simulink model "Quadcopter_CTC_Quaternion_Control"  (R2025a)
settings: Solver=FixedStepAuto  StartTime=0  StopTime=30  FixedStep=step_size  RelTol=1e-5
values from neighbouring files (symbols this model uses):
  g = 9.81    [Parameters.m]
  mQ = 1.5    [Parameters.m]
libraries: aerolibutil x1, sharedutil x1, slpidlib x1
settings Model: Creator=Mohamed Eid  LastModifiedBy=HP
settings DataIOCC: SaveFormat=StructureWithTime
settings OptimizationCC: BlockReduction=off  BufferReuse=off
settings DebuggingCC: SignalInfNanChecking=error  AlgebraicLoopMsg=none
settings ModelReferenceCC: EnableRefExpFcnMdlSchedulingChecks=on
settings RTWCC: GPUComputeCapability=3.5  DLArmComputeVersion=19.05

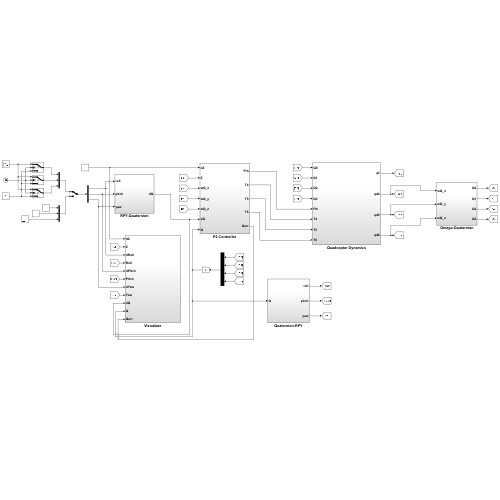
[thumbnail: Simulink's stored preview of the top-level diagram]
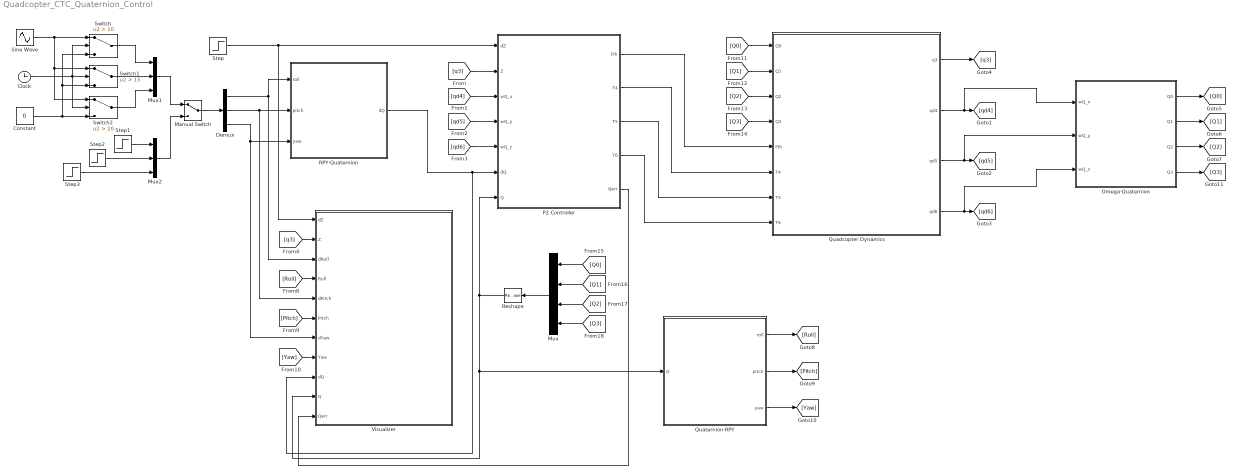
== system Quadcopter_CTC_Quaternion_Control ==
  Clock : Clock
  Constant : Constant  Value=0
  Demux : Demux  Outputs=3
  Manual Switch : ManualSwitch
  Mux : Mux
  Mux1 : Mux  Inputs=3
  Mux2 : Mux  Inputs=3
  Omega-Quaternion : Subsystem
  P2 Controller : Subsystem
  Quadcopter Dynamics : Subsystem
  Quaternion-RPY : Subsystem
  RPY-Quaternion : Subsystem
  Reshape : Reshape  OutputDimensionality=Customize  OutputDimensions=[4,1]
  Sine Wave : Sin  Amplitude=0.5  Frequency=2*pi/5  SampleTime=0
  Step : Step  After=10  SampleTime=0
  Step1 : Step  Time=10  After=30*pi/180  SampleTime=0
  Step2 : Step  Time=15  After=30*pi/180  SampleTime=0
  Step3 : Step  Time=20  After=30*pi/180  SampleTime=0
  Switch : Switch  Criteria=u2 > Threshold  Threshold=10  SaturateOnIntegerOverflow=off  InputSameDT=off
  Switch1 : Switch  Criteria=u2 > Threshold  Threshold=15  SaturateOnIntegerOverflow=off  InputSameDT=off
  Switch2 : Switch  Criteria=u2 > Threshold  Threshold=20  SaturateOnIntegerOverflow=off  InputSameDT=off
  Visualizer : Subsystem
  wires:
  Demux/2 -> Visualizer/5(dPitch), RPY-Quaternion/2(pitch)
  Quadcopter Dynamics/4(qd6) -> Omega-Quaternion/3(wQ_z), [qd6]
  Demux/1 -> RPY-Quaternion/1(roll), Visualizer/3(dRoll)
  Quadcopter Dynamics/2(qd4) -> Omega-Quaternion/1(wQ_x), [qd4]
  Quadcopter Dynamics/3(qd5) -> Omega-Quaternion/2(wQ_y), [qd5]
  Demux/3 -> Visualizer/7(dYaw), RPY-Quaternion/3(yaw)
  Quadcopter Dynamics/1(q3) -> [q3]
  [q3] -> P2 Controller/2(Z)
  [qd6] -> P2 Controller/5(wQ_z)
  [qd5] -> P2 Controller/4(wQ_y)
  [qd4] -> P2 Controller/3(wQ_x)
  Step/1 -> Visualizer/1(dZ), P2 Controller/1(dZ)
  RPY-Quaternion/1(dQ) -> Visualizer/9(dQ), P2 Controller/6(dQ)
  [q3] -> Visualizer/2(Z)
  Mux/1 -> Reshape/1
  Quaternion-RPY/2(pitch) -> [Pitch]
  Quaternion-RPY/1(roll) -> [Roll]
  Quaternion-RPY/3(yaw) -> [Yaw]
  [Roll] -> Visualizer/4(Roll)
  [Pitch] -> Visualizer/6(Pitch)
  [Yaw] -> Visualizer/8(Yaw)
  Reshape/1 -> P2 Controller/7(Q), Visualizer/10(Q), Quaternion-RPY/1(Q)
  P2 Controller/4(T6) -> Quadcopter Dynamics/8(T6)
  P2 Controller/3(T5) -> Quadcopter Dynamics/7(T5)
  P2 Controller/2(T4) -> Quadcopter Dynamics/6(T4)
  P2 Controller/1(Fth) -> Quadcopter Dynamics/5(Fth)
  P2 Controller/5(Qerr) -> Visualizer/11(Qerr)
  Omega-Quaternion/1(Q0) -> [Q0]
  Omega-Quaternion/2(Q1) -> [Q1]
  Omega-Quaternion/3(Q2) -> [Q2]
  Omega-Quaternion/4(Q3) -> [Q3]
  [Q0] -> Quadcopter Dynamics/1(Q0)
  [Q1] -> Quadcopter Dynamics/2(Q1)
  [Q2] -> Quadcopter Dynamics/3(Q2)
  [Q3] -> Quadcopter Dynamics/4(Q3)
  [Q0] -> Mux/1
  [Q1] -> Mux/2
  [Q2] -> Mux/3
  [Q3] -> Mux/4
  Constant/1 -> Switch/3, Switch1/3, Switch2/3
  Sine Wave/1 -> Switch2/1, Switch1/1, Switch/1
  Clock/1 -> Switch2/2, Switch/2, Switch1/2
  Step1/1 -> Mux2/1
  Step2/1 -> Mux2/2
  Step3/1 -> Mux2/3
  Switch1/1 -> Mux1/2
  Switch/1 -> Mux1/1
  Switch2/1 -> Mux1/3
  Manual Switch/1 -> Demux/1
  Mux1/1 -> Manual Switch/1
  Mux2/1 -> Manual Switch/2

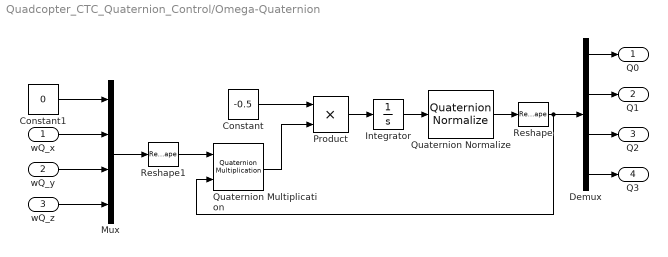
== system Quadcopter_CTC_Quaternion_Control/Omega-Quaternion ==
  wQ_x : Inport
  wQ_y : Inport  Port=2
  wQ_z : Inport  Port=3
  Constant : Constant  Value=-0.5
  Constant1 : Constant  Value=0
  Demux : Demux
  Integrator : Integrator  InitialCondition=[1;0;0;0]
  Mux : Mux
  Product : Product
  Quaternion Multiplication : aerolibutil/Quaternion Multiplication
  Quaternion Normalize : sharedutil/Quaternion Normalize  aMode=aMode
  Reshape : Reshape  OutputDimensionality=Customize  OutputDimensions=[4,1]
  Reshape1 : Reshape  OutputDimensionality=Customize  OutputDimensions=[4,1]
  Q0 : Outport
  Q1 : Outport  Port=2
  Q2 : Outport  Port=3
  Q3 : Outport  Port=4
  wires:
  Integrator/1 -> Quaternion Normalize/1
  Quaternion Normalize/1 -> Reshape/1
  Reshape/1 -> Quaternion Multiplication/2, Demux/1
  Demux/4 -> Q3/1
  Demux/3 -> Q2/1
  Demux/2 -> Q1/1
  Demux/1 -> Q0/1
  Constant/1 -> Product/1
  Quaternion Multiplication/1 -> Product/2
  Product/1 -> Integrator/1
  wQ_z/1 -> Mux/4
  wQ_y/1 -> Mux/3
  wQ_x/1 -> Mux/2
  Constant1/1 -> Mux/1
  Mux/1 -> Reshape1/1
  Reshape1/1 -> Quaternion Multiplication/1

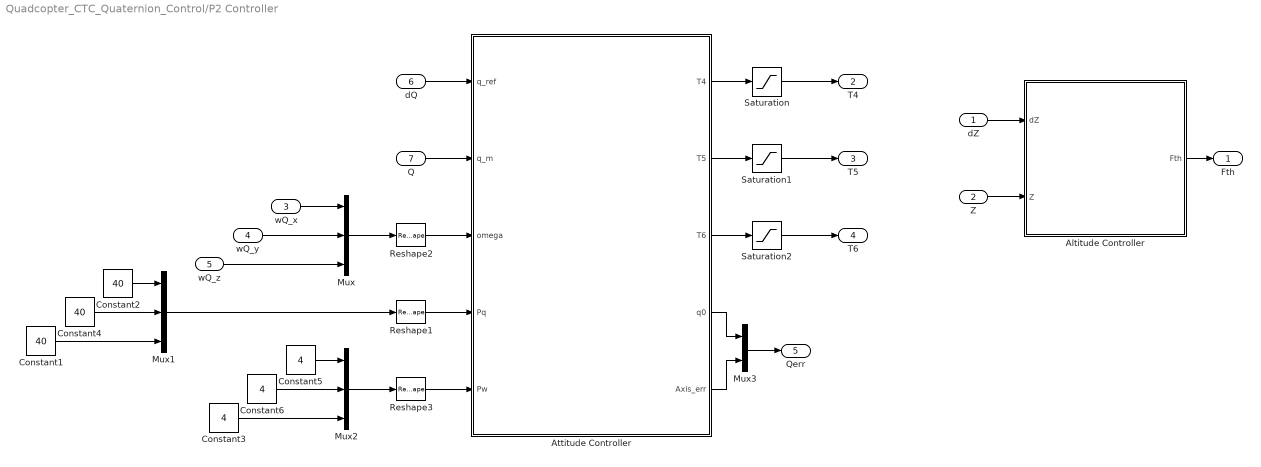
== system Quadcopter_CTC_Quaternion_Control/P2 Controller ==
  dZ : Inport
  Z : Inport  Port=2
  wQ_x : Inport  Port=3
  wQ_y : Inport  Port=4
  wQ_z : Inport  Port=5
  dQ : Inport  Port=6
  Q : Inport  Port=7
  Altitude Controller : Subsystem
  Attitude Controller : MATLAB Function  TreatAsAtomicUnit=on
  Constant1 : Constant  Value=40
  Constant2 : Constant  Value=40
  Constant3 : Constant  Value=4
  Constant4 : Constant  Value=40
  Constant5 : Constant  Value=4
  Constant6 : Constant  Value=4
  Mux : Mux  Inputs=3
  Mux1 : Mux  Inputs=3
  Mux2 : Mux  Inputs=3
  Mux3 : Mux  Inputs=2
  Reshape1 : Reshape  OutputDimensionality=Customize  OutputDimensions=[1,3]
  Reshape2 : Reshape  OutputDimensionality=Customize  OutputDimensions=[3,1]
  Reshape3 : Reshape  OutputDimensionality=Customize  OutputDimensions=[1,3]
  Saturation : Saturate  UpperLimit=1.842326154870013  LowerLimit=-1.842326154870013
  Saturation1 : Saturate  UpperLimit=1.842326154870013  LowerLimit=-1.842326154870013
  Saturation2 : Saturate  UpperLimit=0.104069495295931  LowerLimit=-0.104069495295931
  Fth : Outport
  T4 : Outport  Port=2
  T5 : Outport  Port=3
  T6 : Outport  Port=4
  Qerr : Outport  Port=5
  wires:
  Mux/1 -> Reshape2/1
  wQ_x/1 -> Mux/1
  wQ_y/1 -> Mux/2
  wQ_z/1 -> Mux/3
  Attitude Controller/1(T4) -> Saturation/1
  dZ/1 -> Altitude Controller/1(dZ)
  Z/1 -> Altitude Controller/2(Z)
  Altitude Controller/1(Fth) -> Fth/1
  dQ/1 -> Attitude Controller/1(q_ref)
  Q/1 -> Attitude Controller/2(q_m)
  Reshape2/1 -> Attitude Controller/3(omega)
  Mux3/1 -> Qerr/1
  Attitude Controller/2(T5) -> Saturation1/1
  Attitude Controller/3(T6) -> Saturation2/1
  Attitude Controller/4(q0) -> Mux3/1
  Attitude Controller/5(Axis_err) -> Mux3/2
  Saturation/1 -> T4/1
  Saturation1/1 -> T5/1
  Saturation2/1 -> T6/1
  Constant4/1 -> Mux1/2
  Mux1/1 -> Reshape1/1
  Constant1/1 -> Mux1/3
  Constant2/1 -> Mux1/1
  Constant5/1 -> Mux2/1
  Constant3/1 -> Mux2/3
  Constant6/1 -> Mux2/2
  Mux2/1 -> Reshape3/1
  Reshape1/1 -> Attitude Controller/4(Pq)
  Reshape3/1 -> Attitude Controller/5(Pw)

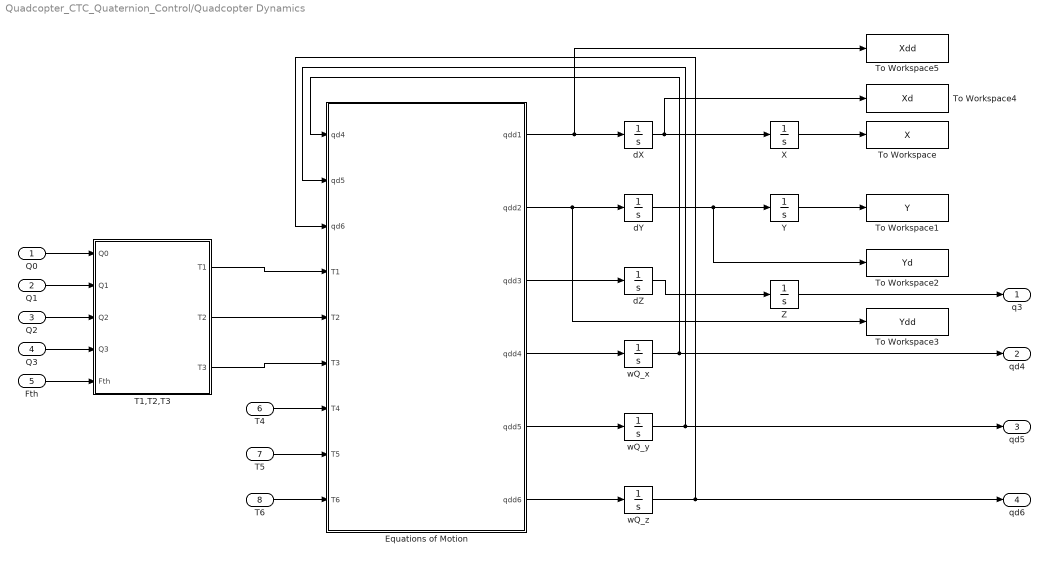
== system Quadcopter_CTC_Quaternion_Control/Quadcopter Dynamics ==
  Q0 : Inport
  Q1 : Inport  Port=2
  Q2 : Inport  Port=3
  Q3 : Inport  Port=4
  Fth : Inport  Port=5
  T4 : Inport  Port=6
  T5 : Inport  Port=7
  T6 : Inport  Port=8
  Equations of Motion : MATLAB Function  TreatAsAtomicUnit=on
  T1,T2,T3 : MATLAB Function  TreatAsAtomicUnit=on
  To Workspace : ToWorkspace  VariableName=X  SaveFormat=Timeseries  SampleTime=-1
  To Workspace1 : ToWorkspace  VariableName=Y  SaveFormat=Timeseries  SampleTime=-1
  To Workspace2 : ToWorkspace  VariableName=Yd  SaveFormat=Timeseries  SampleTime=-1
  To Workspace3 : ToWorkspace  VariableName=Ydd  SaveFormat=Timeseries  SampleTime=-1
  To Workspace4 : ToWorkspace  VariableName=Xd  SaveFormat=Timeseries  SampleTime=-1
  To Workspace5 : ToWorkspace  VariableName=Xdd  SaveFormat=Timeseries  SampleTime=-1
  X : Integrator
  Y : Integrator
  Z : Integrator  LimitOutput=on  LowerSaturationLimit=0
  dX : Integrator
  dY : Integrator
  dZ : Integrator
  wQ_x : Integrator
  wQ_y : Integrator
  wQ_z : Integrator
  q3 : Outport
  qd4 : Outport  Port=2
  qd5 : Outport  Port=3
  qd6 : Outport  Port=4
  wires:
  Equations of Motion/1(qdd1) -> To Workspace5/1, dX/1
  dX/1 -> X/1, To Workspace4/1
  X/1 -> To Workspace/1
  Y/1 -> To Workspace1/1
  dY/1 -> To Workspace2/1, Y/1
  Equations of Motion/2(qdd2) -> To Workspace3/1, dY/1
  Equations of Motion/3(qdd3) -> dZ/1
  dZ/1 -> Z/1
  Z/1 -> q3/1
  Equations of Motion/4(qdd4) -> wQ_x/1
  Equations of Motion/5(qdd5) -> wQ_y/1
  wQ_y/1 -> Equations of Motion/2(qd5), qd5/1
  wQ_z/1 -> Equations of Motion/3(qd6), qd6/1
  Equations of Motion/6(qdd6) -> wQ_z/1
  wQ_x/1 -> qd4/1, Equations of Motion/1(qd4)
  Q3/1 -> T1,T2,T3/4(Q3)
  Q2/1 -> T1,T2,T3/3(Q2)
  Q1/1 -> T1,T2,T3/2(Q1)
  Q0/1 -> T1,T2,T3/1(Q0)
  Fth/1 -> T1,T2,T3/5(Fth)
  T4/1 -> Equations of Motion/7(T4)
  T5/1 -> Equations of Motion/8(T5)
  T6/1 -> Equations of Motion/9(T6)
  T1,T2,T3/2(T2) -> Equations of Motion/5(T2)
  T1,T2,T3/1(T1) -> Equations of Motion/4(T1)
  T1,T2,T3/3(T3) -> Equations of Motion/6(T3)

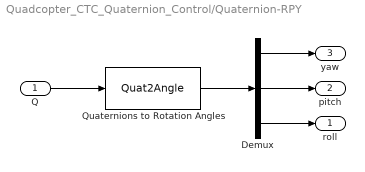
== system Quadcopter_CTC_Quaternion_Control/Quaternion-RPY ==
  Q : Inport
  Demux : Demux  Outputs=3
  Quaternions to Rotation Angles : Quat2Angle
      settings: AttributesFormatString=Rotation Order: %<rotationOrder>
  roll : Outport
  pitch : Outport  Port=2
  yaw : Outport  Port=3
  wires:
  Q/1 -> Quaternions to Rotation Angles/1
  Quaternions to Rotation Angles/1 -> Demux/1
  Demux/2 -> pitch/1
  Demux/3 -> roll/1
  Demux/1 -> yaw/1

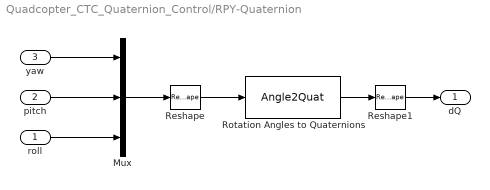
== system Quadcopter_CTC_Quaternion_Control/RPY-Quaternion ==
  roll : Inport
  pitch : Inport  Port=2
  yaw : Inport  Port=3
  Mux : Mux  Inputs=3
  Reshape : Reshape  OutputDimensionality=Customize  OutputDimensions=[1,3]
  Reshape1 : Reshape  OutputDimensionality=Customize  OutputDimensions=[4,1]
  Rotation Angles to Quaternions : Angle2Quat
      settings: AttributesFormatString=Rotation Order: %<rotationOrder>
  dQ : Outport
  wires:
  Rotation Angles to Quaternions/1 -> Reshape1/1
  Mux/1 -> Reshape/1
  Reshape/1 -> Rotation Angles to Quaternions/1
  Reshape1/1 -> dQ/1
  pitch/1 -> Mux/2
  roll/1 -> Mux/3
  yaw/1 -> Mux/1

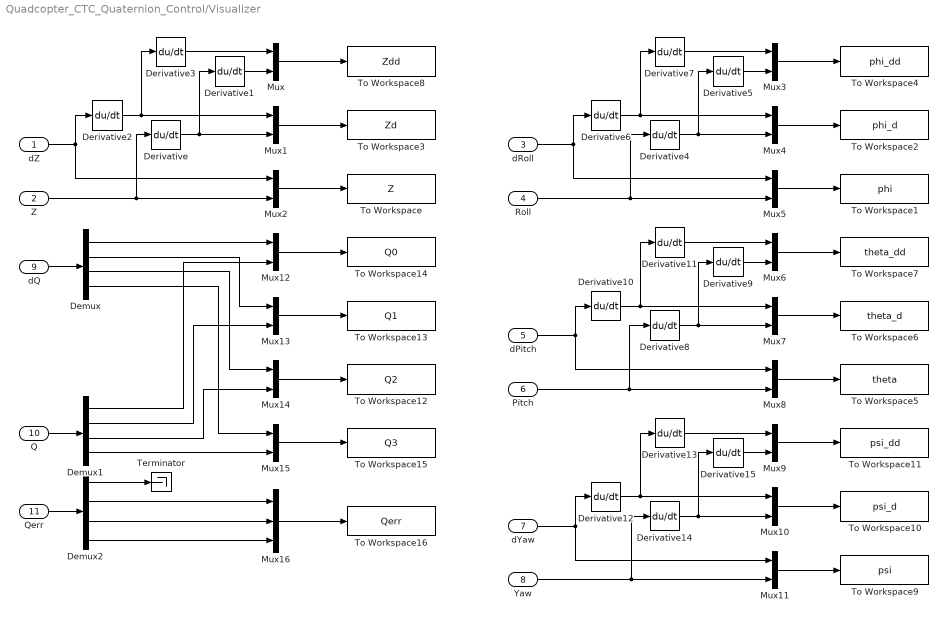
== system Quadcopter_CTC_Quaternion_Control/Visualizer ==
  dZ : Inport
  Z : Inport  Port=2
  dRoll : Inport  Port=3
  Roll : Inport  Port=4
  dPitch : Inport  Port=5
  Pitch : Inport  Port=6
  dYaw : Inport  Port=7
  Yaw : Inport  Port=8
  dQ : Inport  Port=9
  Q : Inport  Port=10
  Qerr : Inport  Port=11
  Demux : Demux
  Demux1 : Demux
  Demux2 : Demux
  Derivative{,1..15} (16 alike) : Derivative
  Mux{,1..15} (16 alike) : Mux  Inputs=2
  Mux16 : Mux  Inputs=3
  Terminator : Terminator
  To Workspace : ToWorkspace  VariableName=Z  SaveFormat=Timeseries  SampleTime=-1
  To Workspace1 : ToWorkspace  VariableName=phi  SaveFormat=Timeseries  SampleTime=-1
  To Workspace10 : ToWorkspace  VariableName=psi_d  SaveFormat=Timeseries  SampleTime=-1
  To Workspace11 : ToWorkspace  VariableName=psi_dd  SaveFormat=Timeseries  SampleTime=-1
  To Workspace12 : ToWorkspace  VariableName=Q2  SaveFormat=Timeseries  SampleTime=-1
  To Workspace13 : ToWorkspace  VariableName=Q1  SaveFormat=Timeseries  SampleTime=-1
  To Workspace14 : ToWorkspace  VariableName=Q0  SaveFormat=Timeseries  SampleTime=-1
  To Workspace15 : ToWorkspace  VariableName=Q3  SaveFormat=Timeseries  SampleTime=-1
  To Workspace16 : ToWorkspace  VariableName=Qerr  SaveFormat=Timeseries  SampleTime=-1
  To Workspace2 : ToWorkspace  VariableName=phi_d  SaveFormat=Timeseries  SampleTime=-1
  To Workspace3 : ToWorkspace  VariableName=Zd  SaveFormat=Timeseries  SampleTime=-1
  To Workspace4 : ToWorkspace  VariableName=phi_dd  SaveFormat=Timeseries  SampleTime=-1
  To Workspace5 : ToWorkspace  VariableName=theta  SaveFormat=Timeseries  SampleTime=-1
  To Workspace6 : ToWorkspace  VariableName=theta_d  SaveFormat=Timeseries  SampleTime=-1
  To Workspace7 : ToWorkspace  VariableName=theta_dd  SaveFormat=Timeseries  SampleTime=-1
  To Workspace8 : ToWorkspace  VariableName=Zdd  SaveFormat=Timeseries  SampleTime=-1
  To Workspace9 : ToWorkspace  VariableName=psi  SaveFormat=Timeseries  SampleTime=-1
  wires:
  Mux/1 -> To Workspace8/1
  Derivative3/1 -> Mux/1
  Derivative1/1 -> Mux/2
  Derivative/1 -> Derivative1/1, Mux1/2
  Derivative2/1 -> Derivative3/1, Mux1/1
  Mux1/1 -> To Workspace3/1
  Mux2/1 -> To Workspace/1
  dZ/1 -> Mux2/1, Derivative2/1
  Z/1 -> Derivative/1, Mux2/2
  Mux3/1 -> To Workspace4/1
  Mux4/1 -> To Workspace2/1
  Roll/1 -> Derivative4/1, Mux5/2
  dRoll/1 -> Mux5/1, Derivative6/1
  Mux5/1 -> To Workspace1/1
  Mux6/1 -> To Workspace7/1
  Mux7/1 -> To Workspace6/1
  Mux8/1 -> To Workspace5/1
  dPitch/1 -> Mux8/1, Derivative10/1
  Pitch/1 -> Derivative8/1, Mux8/2
  Mux9/1 -> To Workspace11/1
  Mux10/1 -> To Workspace10/1
  Mux11/1 -> To Workspace9/1
  Yaw/1 -> Derivative14/1, Mux11/2
  dYaw/1 -> Mux11/1, Derivative12/1
  Derivative6/1 -> Mux4/1, Derivative7/1
  Derivative4/1 -> Mux4/2, Derivative5/1
  Derivative7/1 -> Mux3/1
  Derivative5/1 -> Mux3/2
  Derivative9/1 -> Mux6/2
  Derivative11/1 -> Mux6/1
  Derivative8/1 -> Mux7/2, Derivative9/1
  Derivative10/1 -> Mux7/1, Derivative11/1
  Derivative12/1 -> Mux10/1, Derivative13/1
  Derivative14/1 -> Mux10/2, Derivative15/1
  Derivative13/1 -> Mux9/1
  Derivative15/1 -> Mux9/2
  Mux14/1 -> To Workspace12/1
  Mux13/1 -> To Workspace13/1
  Mux12/1 -> To Workspace14/1
  Mux15/1 -> To Workspace15/1
  Demux/1 -> Mux12/1
  Demux1/4 -> Mux15/2
  Demux/2 -> Mux13/1
  Demux/3 -> Mux14/1
  Demux/4 -> Mux15/1
  Demux1/3 -> Mux14/2
  Demux1/2 -> Mux13/2
  Demux1/1 -> Mux12/2
  dQ/1 -> Demux/1
  Q/1 -> Demux1/1
  Mux16/1 -> To Workspace16/1
  Qerr/1 -> Demux2/1
  Demux2/2 -> Mux16/1
  Demux2/3 -> Mux16/2
  Demux2/4 -> Mux16/3
  Demux2/1 -> Terminator/1

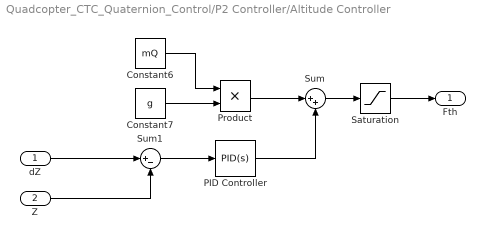
== system Quadcopter_CTC_Quaternion_Control/P2 Controller/Altitude Controller ==
  dZ : Inport
  Z : Inport  Port=2
  Constant6 : Constant  Value=mQ
  Constant7 : Constant  Value=g
  PID Controller : slpidlib/PID Controller  Controller=PID  Form=Parallel  TimeDomain=Continuous-time  UseExternalTs=off  SampleTime=-1  IntegratorMethod=Forward Euler  FilterMethod=Forward Euler  ControllerParametersSource=internal  P=3.93680072164958  I=0.22967015473655  UseKiTs=off  D=14.9935085474605  UseExternalDerivativeSource=off  N=1142.8279760416  UseFilter=on  TunerSelectOption=Transfer Function Based (PID Tuner App)  InitialConditionSource=internal  InitialConditionForIntegrator=0  InitialConditionForFilter=0  DifferentiatorICPrevScaledInput=0  ExternalReset=none  TrackingMode=off  Kt=1  LimitOutput=off  SatLimitsSource=internal  UpperSaturationLimit=inf  LowerSaturationLimit=-inf  LinearizeAsGain=on  AntiWindupMode=none  Kb=1  LimitIntegrator=off  UpperIntegratorSaturationLimit=inf  LowerIntegratorSaturationLimit=-inf  POutMin=[]  POutMax=[]  IOutMin=[]  IOutMax=[]  DOutMin=[]  DOutMax=[]  NOutMin=[]  NOutMax=[]  SumOutMin=[]  SumOutMax=[]  SaturationOutMin=[]  SaturationOutMax=[]  PParamMin=[]  PParamMax=[]  IParamMin=[]  IParamMax=[]  DParamMin=[]  DParamMax=[]  NParamMin=[]  NParamMax=[]  KbParamMin=[]  KbParamMax=[]  KtParamMin=[]  KtParamMax=[]  KbOutMin=[]  KbOutMax=[]  KtOutMin=[]  KtOutMax=[]  IntegratorOutMin=[]  IntegratorOutMax=[]  FilterOutMin=[]  FilterOutMax=[]  SumI1OutMin=[]  SumI1OutMax=[]  SumI2OutMin=[]  SumI2OutMax=[]  SumI3OutMin=[]  SumI3OutMax=[]  SumI4OutMin=[]  SumI4OutMax=[]  SumDOutMin=[]  SumDOutMax=[]  DifferentiatorOutMin=[]  DifferentiatorOutMax=[]  FilterDiffOutCoefMin=[]  FilterDiffOutCoefMax=[]  ReciprocalOutMin=[]  ReciprocalOutMax=[]  SumDenOutMin=[]  SumDenOutMax=[]  SumNumOutMin=[]  SumNumOutMax=[]  DivideOutMin=[]  DivideOutMax=[]  UdiffTsProdOutMin=[]  UdiffTsProdOutMax=[]  NTsProdOutMin=[]  NTsProdOutMax=[]  UintegralTsProdOutMin=[]  UintegralTsProdOutMax=[]  UngainTsProdOutMin=[]  UngainTsProdOutMax=[]  ClampingZeroOutDataTypeStr=Inherit: Inherit via back propagation  ClampingZeroOutMin=[]  ClampingZeroOutMax=[]  FilterDenConstantOutDataTypeStr=Inherit: Inherit via back propagation  FilterDenConstantOutMin=[]  FilterDenConstantOutMax=[]  PCopyOutDataTypeStr=Inherit: Inherit via back propagation  PCopyOutMin=[]  PCopyOutMax=[]  NCopyOutDataTypeStr=Inherit: Inherit via back propagation  NCopyOutMin=[]  NCopyOutMax=[]  IntegratorContinuousStateAttributes=''  IntegratorStateMustResolveToSignalObject=off  IntegratorRTWStateStorageClass=Auto  FilterContinuousStateAttributes=''  FilterStateMustResolveToSignalObject=off  FilterRTWStateStorageClass=Auto  ParallelPVariant=InternalParameters  IdealPVariant=Disabled  IVariant=InternalParameters  DVariant=InternalParameters  IntegratorVariant=Continuous  SatVariant=Disabled  AWVariant=Passthrough  PCopyVariant=Disabled  TRVariant=Disabled  FdbkBlocksVariant=Forward  IdealPFdbkVariant=Disabled  SatFdbkVariant=Disabled  DerivativeFilterVariant=ContFilter  NVariant=InternalParameters  NCopyVariant=Disabled  FilterICVariant=InternalICsFilter  IntegratorICVariant=InternalICs  ExternalResetVariant=Disabled  TRSumVariant=Passthrough  SumFdbkVariant=Disabled  SumVariant=Sum_PID  TsampFilterVariant=InternalTs  TsampNgainVariant=Passthrough  TsampIntegralVariant=Disabled_SignalSpec  ExternalSaturationOutDataTypeStr=Inherit: Same as second input  DerivativeSourceVariant=ErrorSignal  PreIntVariant=InternalPreInt
  Product : Product
  Saturation : Saturate  UpperLimit=23.029076935875167  LowerLimit=0
  Sum : Sum  Inputs=|++
  Sum1 : Sum  Inputs=|+-
  Fth : Outport
  wires:
  Constant6/1 -> Product/1
  Sum1/1 -> PID Controller/1
  dZ/1 -> Sum1/1
  Product/1 -> Sum/1
  Constant7/1 -> Product/2
  PID Controller/1 -> Sum/2
  Z/1 -> Sum1/2
  Sum/1 -> Saturation/1
  Saturation/1 -> Fth/1

== matlab function Quadcopter_CTC_Quaternion_Control/P2 Controller/Attitude Controller ==
  data: q_ref input; T4 output; q_m input; omega input; Pq input; Pw input; T5 output; T6 output; q0 output; Axis_err output
function [T4,T5,T6,q0,Axis_err] = quaternion_attitude_controller(q_ref, q_m, omega, Pq, Pw)
% QUATERNION_ATTITUDE_CONTROLLER
% Implements the full quaternion-based P² attitude controller
% q_ref: desired quaternion [q0; q1; q2; q3]
% q_m: measured quaternion [q0; q1; q2; q3]
% omega: measured angular velocity [wx; wy; wz]
% Pq: proportional gain for quaternion error
% Pomega: proportional gain for angular velocity

% Arrange Pq & Pw
Pq = [Pq(1),0,0;
      0,Pq(2),0;
      0,0,Pq(3)];
Pw = [Pw(1),0,0;
      0,Pw(2),0;
      0,0,Pw(3)];

% === 1) Compute quaternion conjugate ===
q_m_conj = [q_m(1); -q_m(2:4)];

% === 2) Quaternion error: q_err = q_ref ⊗ q_m_conj ===
q_err = quatmultiply(q_ref',q_m_conj');  % MATLAB needs row vectors for quatmultiply
q_err = q_err';  % convert back to column

% === 3) Extract axis error (vector part) ===
Axis_err = q_err(2:4);

% % === 4) Flip axis if q0 < 0 ===
if q_err(1) < 0
    Axis_err = -Axis_err;
end

% === 5) Compute control torque ===
tau = -Pq * Axis_err - Pw * omega;
T4 = tau(1);
T5 = tau(2);
T6 = tau(3);
q0 = q_err(1);

end

== matlab function Quadcopter_CTC_Quaternion_Control/Quadcopter Dynamics/Equations of Motion ==
  data: qd4 input; qd5 input; qd6 input; T1 input; T2 input; qdd1 output; T3 input; T4 input; T5 input; T6 input; qdd2 output; qdd3 output; qdd4 output; qdd5 output; qdd6 output
function [qdd1,qdd2,qdd3,qdd4,qdd5,qdd6] = quadcopter_dynamics(qd4,qd5,qd6,T1,T2,T3,T4,T5,T6)

%Output
qdd1 = 0.6667*T1;
qdd2 = 0.6667*T2;
qdd3 = 0.6667*T3 - 9.81;

wQ = [qd4;qd5;qd6];
IQ = [0.012273,0,0;
      0,0.012526,0;
      0,0,0.020953];

T = [T4;T5;T6];

wQd = IQ\(T - cross(wQ, IQ*wQ));

qdd4 = wQd(1);
qdd5 = wQd(2);
qdd6 = wQd(3);

% qdd4 = (T4 + (0.012526-0.020953)*qd5*qd6)/0.012273;
% qdd5 = (T5 + (0.020953-0.012273)*qd4*qd6)/0.012526;
% qdd6 = (T6 + (0.012273-0.012526)*qd5*qd4)/0.020953;
end

== matlab function Quadcopter_CTC_Quaternion_Control/Quadcopter Dynamics/T1,T2,T3 ==
  data: Q0 input; T1 output; Q1 input; Q2 input; Q3 input; Fth input; T2 output; T3 output
function [T1,T2,T3] = calc_f(Q0,Q1,Q2,Q3,Fth)

% Rotate thrust vector
q = [Q0,Q1,Q2,Q3];
q_conj = [Q0,-Q1,-Q2,-Q3];
F = [0,0,0,Fth];
T = quatmultiply(q_conj,quatmultiply(q,F));

% q0 = Q0;
% qx = Q1;
% qy = Q2;
% qz = Q3;
% 
% R = [1 - 2*qy^2 - 2*qz^2,     2*qx*qy - 2*qz*q0,     2*qx*qz + 2*qy*q0;
%      2*qx*qy + 2*qz*q0, 1 - 2*qx^2 - 2*qz^2,     2*qy*qz - 2*qx*q0;
%      2*qx*qz - 2*qy*q0,     2*qy*qz + 2*qx*q0, 1 - 2*qx^2 - 2*qy^2]
% 
% T = R * [0;0;Fth];

% Output
T1 = T(2);
T2 = T(3);
T3 = T(4);

end
